simulink model "Practical_vs_Ideal_Three_Phase_Transformer"  (R2025a)
settings: Solver=ode23tb  StartTime=0.0  StopTime=0.2  MaxStep=1e-4  RelTol=1e-3
libraries: spsRMSLib x8, spsACVoltageSourceLib x6, spsPower3phInstantaneousLib x4, spsThreePhaseVIMeasurementLib x4, spsGroundLib x2, spsThreePhaseSeriesRLCLoadLib x2, spsThreePhaseTransformerTwoWindingsLib x2, sps_lib x1
settings Model: Creator=Jawad  LastModifiedBy=Jawad

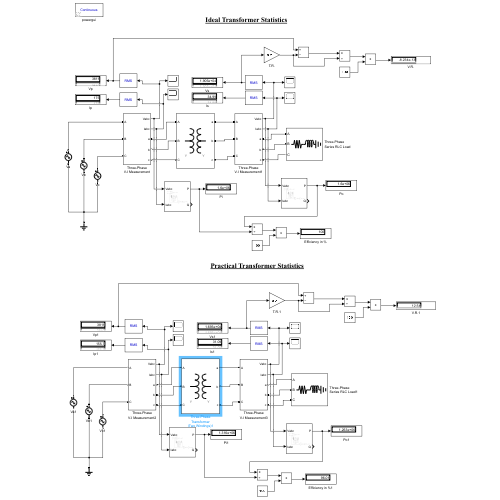
[thumbnail: Simulink's stored preview of the top-level diagram]
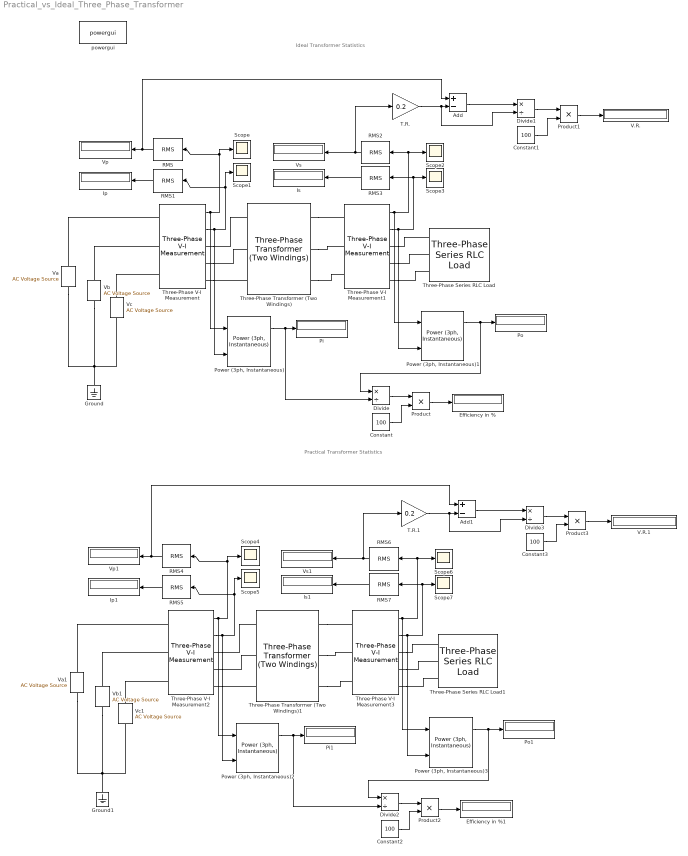
== system Practical_vs_Ideal_Three_Phase_Transformer ==
  note: Ideal Transformer Statistics
  note: Practical Transformer Statistics
  Add : Sum  Inputs=+-
  Add1 : Sum  Inputs=+-
  Constant{,1..3} (4 alike) : Constant  Value=100
  Divide{,1..3} (4 alike) : Product  Inputs=*/
  Efficiency in % : Display
  Efficiency in %1 : Display
  Ground : spsGroundLib/Ground  LConnTagsString=a
  Ground1 : spsGroundLib/Ground  LConnTagsString=a
  Ip : Display
  Ip1 : Display
  Is : Display
  Is1 : Display
  Pi : Display
  Pi1 : Display
  Po : Display
  Po1 : Display
  Power (3ph, Instantaneous){,1..3} (4 alike) : spsPower3phInstantaneousLib/Power (3ph, Instantaneous)
  Product{,1..3} (4 alike) : Product
  RMS{,1..7} (8 alike) : spsRMSLib/RMS  TrueRMS=off  Freq=50  RMSInit=0  Ts=0
  Scope{,1..7} (8 alike) : Scope
      Scope settings: ActiveDisplayYMinimum=-6736.0902871668777  ActiveDisplayYMaximum=6736.0893810743028
      Scope2 settings: DataLoggingVariableName=ScopeData2
      Scope3 settings: ActiveDisplayYMinimum=-1  ActiveDisplayYMaximum=1  DataLoggingVariableName=ScopeData3
      Scope4 settings: ActiveDisplayYMinimum=-6736.0902871668777  ActiveDisplayYMaximum=6736.0893810743028  DataLoggingVariableName=ScopeData4
      Scope5 settings: DataLoggingVariableName=ScopeData5
      Scope6 settings: DataLoggingVariableName=ScopeData6
      Scope7 settings: ActiveDisplayYMinimum=-1  ActiveDisplayYMaximum=1  DataLoggingVariableName=ScopeData7
  T.R. : Gain  Gain=0.2
  T.R.1 : Gain  Gain=0.2
  Three-Phase Series RLC Load : spsThreePhaseSeriesRLCLoadLib/Three-Phase Series RLC Load  LConnTagsString=A|B|C  Configuration=Y (grounded)  NominalVoltage=33e3  Vabc=[1e3 1e3 1e3]  Vabcp=[1e3 1e3 1e3]  NominalFrequency=50  UnbalancedPower=off  ActivePower=1600e3  InductivePower=1200e3  CapacitivePower=0  Pabc=[10e3 9e3 11e3]  QLabc=[100 90 110]  QCabc=[100 90 110]  Pabcp=[10e3 9e3 11e3]  QLabcp=[100 90 110]  QCabcp=[100 90 110]  Measurements=None  LoadType=constant Z
  Three-Phase Series RLC Load1 : spsThreePhaseSeriesRLCLoadLib/Three-Phase Series RLC Load  LConnTagsString=A|B|C  Configuration=Y (grounded)  NominalVoltage=33e3  Vabc=[1e3 1e3 1e3]  Vabcp=[1e3 1e3 1e3]  NominalFrequency=50  UnbalancedPower=off  ActivePower=1600e3  InductivePower=1200e3  CapacitivePower=0  Pabc=[10e3 9e3 11e3]  QLabc=[100 90 110]  QCabc=[100 90 110]  Pabcp=[10e3 9e3 11e3]  QLabcp=[100 90 110]  QCabcp=[100 90 110]  Measurements=None  LoadType=constant Z
  Three-Phase Transformer (Two Windings) : spsThreePhaseTransformerTwoWindingsLib/Three-Phase Transformer (Two Windings)  Winding1Connection=Y  Winding2Connection=Y  CoreType=Three single-phase transformers  SetSaturation=off  Hysteresis=off  DataFile='hysteresis'  SetInitialFlux=off  Measurements=None  UNITS=SI  NominalPower=[ 2000e3 , 50 ]  Winding1=[6.6e3 0 0]  Winding2=[33e3 0 0]  Rm=inf  Lm=inf  L0=0.28887  Saturation=[0 0;0.059382 17.153;24.742 21.728]  InitialFluxes=[11.436 -11.436 10.006]  BreakLoop=off  DiscreteSolver=Trapezoidal iterative  DataType=on  TransfoNumber=1
  Three-Phase Transformer (Two Windings)1 : spsThreePhaseTransformerTwoWindingsLib/Three-Phase Transformer (Two Windings)  Winding1Connection=Y  Winding2Connection=Y  CoreType=Three single-phase transformers  SetSaturation=off  Hysteresis=off  DataFile='hysteresis'  SetInitialFlux=off  Measurements=None  UNITS=SI  NominalPower=[ 2000e3 , 50 ]  Winding1=[6.6e3 0.5 8.27e-3]  Winding2=[33e3 4.3 0.069]  Rm=10000  Lm=500  L0=0.28887  Saturation=[0 0;0.059382 17.153;24.742 21.728]  InitialFluxes=[11.436 -11.436 10.006]  BreakLoop=off  DiscreteSolver=Trapezoidal iterative  DataType=on  TransfoNumber=1
  Three-Phase V-I Measurement{,1..3} (4 alike) : spsThreePhaseVIMeasurementLib/Three-Phase V-I Measurement  VoltageMeasurement=phase-to-ground  SetLabelV=off  LabelV=Vabc  Vpu=off  VpuLL=off  CurrentMeasurement=yes  SetLabelI=off  LabelI=Iabc  Ipu=off  Pbase=100e6  Vbase=500e3  OutputType=Complex  PhasorSimulation=off  PSBequivalent=0
  V.R. : Display
  V.R.1 : Display
  Va : spsACVoltageSourceLib/AC Voltage Source  Amplitude=(6.6e3*sqrt(2))/sqrt(3)  Phase=0  Frequency=50  SampleTime=0  Measurements=None  BusType=swing  Pref=10e3  Qref=0  Qmin=-inf  Qmax=+inf
  Va1 : spsACVoltageSourceLib/AC Voltage Source  Amplitude=(6.6e3*sqrt(2))/sqrt(3)  Phase=0  Frequency=50  SampleTime=0  Measurements=None  BusType=swing  Pref=10e3  Qref=0  Qmin=-inf  Qmax=+inf
  Vb : spsACVoltageSourceLib/AC Voltage Source  Amplitude=(6.6e3*sqrt(2))/sqrt(3)  Phase=-120  Frequency=50  SampleTime=0  Measurements=None  BusType=swing  Pref=10e3  Qref=0  Qmin=-inf  Qmax=+inf
  Vb1 : spsACVoltageSourceLib/AC Voltage Source  Amplitude=(6.6e3*sqrt(2))/sqrt(3)  Phase=-120  Frequency=50  SampleTime=0  Measurements=None  BusType=swing  Pref=10e3  Qref=0  Qmin=-inf  Qmax=+inf
  Vc : spsACVoltageSourceLib/AC Voltage Source  Amplitude=(6.6e3*sqrt(2))/sqrt(3)  Phase=120  Frequency=50  SampleTime=0  Measurements=None  BusType=swing  Pref=10e3  Qref=0  Qmin=-inf  Qmax=+inf
  Vc1 : spsACVoltageSourceLib/AC Voltage Source  Amplitude=(6.6e3*sqrt(2))/sqrt(3)  Phase=120  Frequency=50  SampleTime=0  Measurements=None  BusType=swing  Pref=10e3  Qref=0  Qmin=-inf  Qmax=+inf
  Vp : Display
  Vp1 : Display
  Vs : Display
  Vs1 : Display
  powergui : sps_lib/powergui  Priority=1  SimulationMode=Continuous  SampleTime=50e-6  frequency=60  Iterations=50  frequencyindice=50  Pbase=100e6  ErrMax=1e-4  UnitsV=kV  UnitsW=MW  buscounter=0  FunctionMessages=off  echomessages=off  EnableUseOfTLC=off  CurrentSourceSwitches=off  DisableSnubberDevices=off  DisableRonSwitches=off  DisableVfSwitches=off  DisplayEquations=off  AutomaticDiscreteSolvers=off  SolverType=Tustin/Backward Euler (TBE)  Interpol=off  ExternalGateDelay=off  methode=off  Ts=100  x0status=blocks  SPID=on  SwTol=0  HookPort=off  NonlinearTolerance=1e-4  nMaxIteration=100  ContinueOnMaxIteration=off  RestoreLinks=warning  ResistiveCurrentMeasurement=off  Frange=[0:2:500]  Ylog=off  Xlog=on  ShowGrid=off  save=off  variable=ZData  structure=0  ZoomFFT=off  StartTime=0.0  cycles=1  DisplayStyle=1  fundamental=60  FreqAxis=off  MaxFrequency=1000  frequencyindicesteady=1  RmsSteady=1  display=off
  wires:
  RMS2/1 -> T.R./1, Vs/1
  Three-Phase V-I Measurement1/1 -> "Power (3ph, Instantaneous)1"/1, Scope2/1, RMS2/1
  RMS1/1 -> Ip/1
  Three-Phase V-I Measurement/2 -> "Power (3ph, Instantaneous)"/2, Scope1/1, RMS1/1
  Three-Phase V-I Measurement/1 -> "Power (3ph, Instantaneous)"/1, Scope/1, RMS/1
  RMS3/1 -> Is/1
  RMS/1 -> Add/1, Vp/1
  Three-Phase V-I Measurement1/2 -> "Power (3ph, Instantaneous)1"/2, Scope3/1, RMS3/1
  "Power (3ph, Instantaneous)"/1 -> Divide/2, Pi/1
  "Power (3ph, Instantaneous)1"/1 -> Divide/1, Po/1
  Divide/1 -> Product/1
  Constant/1 -> Product/2
  Product/1 -> Efficiency in %/1
  T.R./1 -> Divide1/2, Add/2
  Add/1 -> Divide1/1
  Divide1/1 -> Product1/1
  Constant1/1 -> Product1/2
  Product1/1 -> V.R./1
  T.R.1/1 -> Divide3/2, Add1/2
  Product2/1 -> Efficiency in %1/1
  RMS4/1 -> Add1/1, Vp1/1
  RMS7/1 -> Is1/1
  RMS6/1 -> T.R.1/1, Vs1/1
  Constant2/1 -> Product2/2
  Three-Phase V-I Measurement3/1 -> "Power (3ph, Instantaneous)3"/1, Scope6/1, RMS6/1
  RMS5/1 -> Ip1/1
  Three-Phase V-I Measurement2/2 -> "Power (3ph, Instantaneous)2"/2, Scope5/1, RMS5/1
  "Power (3ph, Instantaneous)2"/1 -> Divide2/2, Pi1/1
  Three-Phase V-I Measurement3/2 -> "Power (3ph, Instantaneous)3"/2, Scope7/1, RMS7/1
  "Power (3ph, Instantaneous)3"/1 -> Divide2/1, Po1/1
  Constant3/1 -> Product3/2
  Product3/1 -> V.R.1/1
  Divide2/1 -> Product2/1
  Add1/1 -> Divide3/1
  Divide3/1 -> Product3/1
  Three-Phase V-I Measurement2/1 -> "Power (3ph, Instantaneous)2"/1, Scope4/1, RMS4/1
  connections:
  Vc/LConn1 -- Ground/LConn1 -- Va/LConn1 -- Vb/LConn1
  Three-Phase V-I Measurement1/RConn1 -- Three-Phase Series RLC Load/LConn1
  Va/RConn1 -- Three-Phase V-I Measurement/LConn1
  Three-Phase Transformer (Two Windings)/RConn3 -- Three-Phase V-I Measurement1/LConn3
  Three-Phase Transformer (Two Windings)/RConn1 -- Three-Phase V-I Measurement1/LConn1
  Three-Phase Transformer (Two Windings)/RConn2 -- Three-Phase V-I Measurement1/LConn2
  Three-Phase V-I Measurement1/RConn2 -- Three-Phase Series RLC Load/LConn2
  Three-Phase V-I Measurement/RConn3 -- Three-Phase Transformer (Two Windings)/LConn3
  Three-Phase V-I Measurement1/RConn3 -- Three-Phase Series RLC Load/LConn3
  Vc/RConn1 -- Three-Phase V-I Measurement/LConn3
  Vb/RConn1 -- Three-Phase V-I Measurement/LConn2
  Three-Phase V-I Measurement/RConn1 -- Three-Phase Transformer (Two Windings)/LConn1
  Three-Phase V-I Measurement/RConn2 -- Three-Phase Transformer (Two Windings)/LConn2
  Vc1/LConn1 -- Ground1/LConn1 -- Va1/LConn1 -- Vb1/LConn1
  Three-Phase Transformer (Two Windings)1/RConn1 -- Three-Phase V-I Measurement3/LConn1
  Vb1/RConn1 -- Three-Phase V-I Measurement2/LConn2
  Three-Phase V-I Measurement2/RConn1 -- Three-Phase Transformer (Two Windings)1/LConn1
  Three-Phase V-I Measurement2/RConn2 -- Three-Phase Transformer (Two Windings)1/LConn2
  Three-Phase V-I Measurement3/RConn3 -- Three-Phase Series RLC Load1/LConn3
  Three-Phase V-I Measurement2/RConn3 -- Three-Phase Transformer (Two Windings)1/LConn3
  Three-Phase Transformer (Two Windings)1/RConn2 -- Three-Phase V-I Measurement3/LConn2
  Three-Phase V-I Measurement3/RConn1 -- Three-Phase Series RLC Load1/LConn1
  Three-Phase V-I Measurement3/RConn2 -- Three-Phase Series RLC Load1/LConn2
  Three-Phase Transformer (Two Windings)1/RConn3 -- Three-Phase V-I Measurement3/LConn3
  Va1/RConn1 -- Three-Phase V-I Measurement2/LConn1
  Vc1/RConn1 -- Three-Phase V-I Measurement2/LConn3
